simulink model "RSlatch_simfile"  (Simulink 7.2)
settings: Solver=VariableStepDiscrete  StartTime=0.0  StopTime=100.0  RelTol=1e-3
settings Model: Creator=mweeks  LastModifiedBy=mweeks  BufferReuse=off
settings OptimizationCC: BlockReduction=off  OptimizeBlockIOStorage=off  BufferReuse=off  ExpressionFolding=off  LocalBlockOutputs=off
settings DebuggingCC: InheritedTsInSrcMsg=none  DiscreteInheritContinuousMsg=none  StrictBusMsg=ErrorLevel1

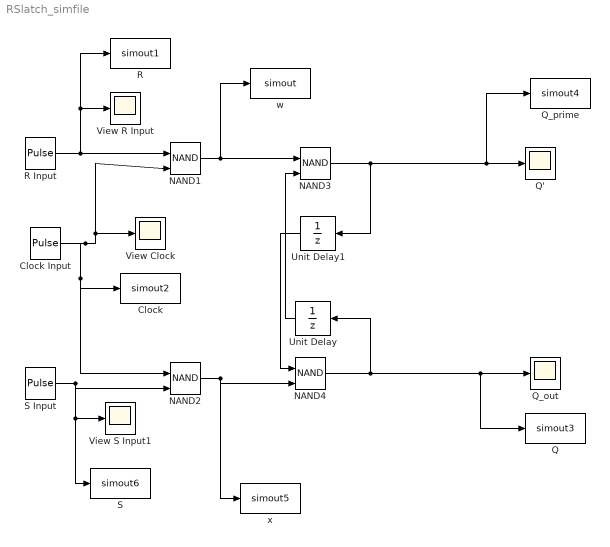
== system RSlatch_simfile ==
  Clock : ToWorkspace  VariableName=simout2  SampleTime=-1  SaveFormat=Structure
  Clock Input : DiscretePulseGenerator  PulseType=Time based  Period=10  PulseWidth=50  PhaseDelay=5
  NAND1 : Logic  Operator=NAND  IconShape=distinctive  AllPortsSameDT=off  SampleTime=0.1
  NAND2 : Logic  Operator=NAND  IconShape=distinctive  AllPortsSameDT=off  SampleTime=0.1
  NAND3 : Logic  Operator=NAND  IconShape=distinctive  AllPortsSameDT=off  SampleTime=0.1
  NAND4 : Logic  Operator=NAND  IconShape=distinctive  AllPortsSameDT=off  OutDataTypeMode=boolean  OutDataTypeStr=boolean
  Q : ToWorkspace  VariableName=simout3  SampleTime=-1  SaveFormat=Structure
  Q' : Scope
      settings: TimeRange=10
  Q_out : Scope
      settings: SaveName=ScopeData3
  Q_prime : ToWorkspace  VariableName=simout4  SampleTime=-1  SaveFormat=Structure
  R : ToWorkspace  VariableName=simout1  SampleTime=-1  SaveFormat=Structure
  R Input : DiscretePulseGenerator  PulseType=Time based  Period=30  PulseWidth=50
  S : ToWorkspace  VariableName=simout6  SampleTime=-1  SaveFormat=Structure
  S Input : DiscretePulseGenerator  PulseType=Time based  Period=60  PulseWidth=50  PhaseDelay=25
  Unit Delay : UnitDelay  Orientation=left
  Unit Delay1 : UnitDelay  Orientation=left
  View Clock : Scope
  View R Input : Scope
      settings: TimeRange=10  SaveName=ScopeData2
  View S Input1 : Scope
      settings: TimeRange=10  SaveName=ScopeData4
  w : ToWorkspace  VariableName=simout  SampleTime=-1  SaveFormat=Structure
  x : ToWorkspace  VariableName=simout5  SampleTime=-1  SaveFormat=Structure
  wires:
  R Input/1 -> View R Input/1, R/1, NAND1/1
  NAND1/1 -> w/1, NAND3/1
  NAND2/1 -> x/1, NAND4/2
  NAND3/1 -> Q'/1, Q_prime/1, Unit Delay1/1
  NAND4/1 -> Q_out/1, Q/1, Unit Delay/1
  Unit Delay1/1 -> NAND4/1
  Unit Delay/1 -> NAND3/2
  S Input/1 -> NAND2/2, View S Input1/1, S/1
  Clock Input/1 -> Clock/1, NAND2/1, NAND1/2, View Clock/1
